simulink model "sl_ControlRobotReal_RRR"  (R2016b)
settings: Solver=ode45  StartTime=0.0  StopTime=t_sim  MaxStep=1e-3  RelTol=1e-3  EnableMultiTasking=on
values from neighbouring files (symbols this model uses):
  Kp1 = 1652.2*Ti1    (= 594.792)    [controladorPID.m]
  Kp2 = 5227.8*Ti2    (= 2091.12)    [controladorPID.m]
  Kp3 = 2761.4*Ti3    (= 994.104)    [controladorPID.m]
  n_ptos = 4    [pruebasCONTROL.m]
  R1 = 50    [modDinamico_Inverso_Ideal_CR.m]    (also in modDinamico_Inverso_Ideal_SR.m = 1; modDinamico_Inverso_Real_CR.m; modDinamico_Inverso_Real_SR.m = 1; pruebasCONTROL.m = 1)
  R2 = 30    [modDinamico_Inverso_Ideal_CR.m]    (also in modDinamico_Inverso_Ideal_SR.m = 1; modDinamico_Inverso_Real_CR.m; modDinamico_Inverso_Real_SR.m = 1; pruebasCONTROL.m = 1)
  R3 = 15    [modDinamico_Inverso_Ideal_CR.m]    (also in modDinamico_Inverso_Ideal_SR.m = 1; modDinamico_Inverso_Real_CR.m; modDinamico_Inverso_Real_SR.m = 1; pruebasCONTROL.m = 1)
  t_init_tray = 2    [pruebasCONTROL.m]
  t_mov = 1    [pruebasCONTROL.m]
  Td1 = (0.18^2)/(0.18*2)    (= 0.09)    [controladorPID.m]
  Td2 = (0.2^2)/(0.2*2)    (= 0.1)    [controladorPID.m]
  Td3 = (0.18^2)/(0.18*2)    (= 0.09)    [controladorPID.m]
  Ti1 = 2*0.18    (= 0.36)    [controladorPID.m]
  Ti2 = 2*0.2    (= 0.4)    [controladorPID.m]
  Ti3 = 2*0.18    (= 0.36)    [controladorPID.m]
  Tm = 0.001    [controladorPD.m]    (also in pruebasCONTROL.m)
  XYZ_fin = CinematicaDirecta([pi/2;pi/3;-pi/3])    [pruebasCONTROL.m]
  XYZ_init = CinematicaDirecta([q1_init;q2_init;q3_init])    [pruebasCONTROL.m]
undefined symbols (not defined in the file or in its folder): XYZ_med
undefined symbols (not defined in the file): q1_init, q2_init, q3_init
settings Model: ExtModeTrigMode=oneshot  ExtModeArmWhenConnect=off  Creator=mortega  LastModifiedBy=marrcogrova
settings DataIOCC: SaveFormat=Array  SignalLoggingSaveFormat=ModelDataLogs
settings OptimizationCC: BlockReduction=off  BooleanDataType=off  ExpressionDepthLimit=2147483647  InitFltsAndDblsToZero=on  LifeSpan=inf
settings DebuggingCC: SaveWithParameterizedLinksMsg=none  UnderspecifiedInitializationDetection=Classic  MergeDetectMultiDrivingBlocksExec=none  SignalResolutionControl=TryResolveAllWithWarning  MultiTaskDSMMsg=warning  MultiTaskCondExecSysMsg=none  FcnCallInpInsideContextMsg=warning  StateNameClashWarn=warning  SFUnexpectedBacktrackingDiag=warning  SFNoUnconditionalDefaultTransitionDiag=warning  SFExecutionAtInitializationDiag=none
settings HardwareCC: ProdBitPerPointer=32  ProdBitPerSizeT=32  ProdBitPerPtrDiffT=32  ProdLargestAtomicFloat=None  ProdIntDivRoundTo=Undefined  ProdEndianess=Unspecified  ProdWordSize=32  ProdHWDeviceType=32-bit Generic  TargetBitPerLong=64  TargetBitPerPointer=64  TargetBitPerSizeT=64  TargetBitPerPtrDiffT=64  TargetLongLongMode=on  TargetIntDivRoundTo=Zero  TargetEndianess=LittleEndian  TargetWordSize=64  TargetHWDeviceType=MATLAB Host  ProdEqTarget=off
settings ModelReferenceCC: PropagateSignalLabelsOutOfModel=off
settings GRTTargetCC: TargetFcnLib=ansi_tfl_tmw.mat  TargetLangStandard=C89/C90 (ANSI)  CombineOutputUpdateFcns=off  GRTInterface=on
settings ConfigComp: CovMetricSettings=dw  CovHtmlReporting=on  CovSaveCumulativeToWorkspaceVar=on  CovSaveSingleToWorkspaceVar=on  CovExternalEMLEnable=off

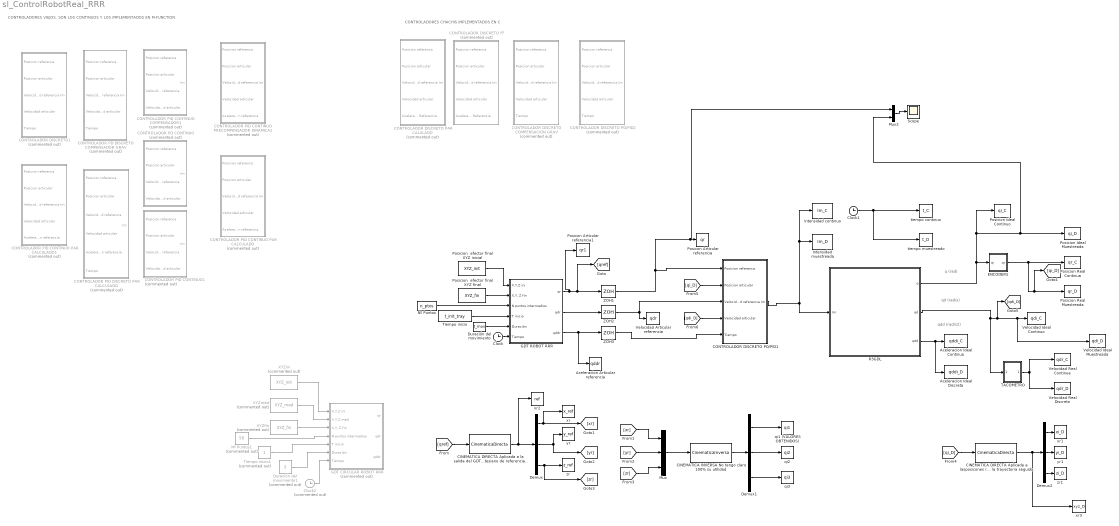
== system sl_ControlRobotReal_RRR ==
  note: CONTROLADORES VIEJOS.
      | SON LOS CONTINUOS Y LOS IMPLEMENTADOS EN M-FUNCTION
  note: q (rad)
  note: qd (rad/s)
  note: qdd (rad/s2)
  note: CONTROLADORES CHACHIS IMPLEMENTADOS EN C
  Aceleracion Articular referencia : ToWorkspace  VariableName=qddr  SampleTime=Tm
  Aceleracion Ideal Continua : ToWorkspace  VariableName=qddi_C  SampleTime=-1
  Aceleracion Ideal Discreta : ToWorkspace  VariableName=qddi_D  SampleTime=Tm
  CINEMATICA DIRECTA Aplicada a la salida del GDT para conocer la trayectoria en el plano cartesiano de referencia.. : MATLABFcn  MATLABFcn=CinematicaDirecta  OutputDimensions=3
  CINEMATICA DIRECTA Aplicada a lasposicones recogidas del robot para concer la trayectoria seguida. : MATLABFcn  MATLABFcn=CinematicaDirecta  OutputDimensions=3
  CINEMATICA INVERSA No tengo claro 100% su utilidad : MATLABFcn  MATLABFcn=CinematicaInversa  OutputDimensions=3
  CONTROLADOR DISCRETO COMPENSACION GRAV : Subsystem  Commented=on
  CONTROLADOR DISCRETO FF : Subsystem  Commented=on
  CONTROLADOR DISCRETO PAR CALULADO : Subsystem  Commented=on
  CONTROLADOR DISCRETO PD/PID1 : Subsystem
  CONTROLADOR DISCRETO PD/PID2 : Subsystem  Commented=on
  CONTROLADOR DISCRETO1 : Subsystem  Commented=on
  CONTROLADOR PD CONTINUO : Subsystem  Commented=on
  CONTROLADOR PD DISCRETO COMPENSADOR GRAV : Subsystem  Commented=on
  CONTROLADOR PID CONTINUO COMPENSADOR1 : Subsystem  Commented=on
  CONTROLADOR PID CONTINUO PAR CALCULADO : Subsystem  Commented=on
  CONTROLADOR PID CONTINUO PAR CALCULADO1 : Subsystem  Commented=on
  CONTROLADOR PID CONTINUO PRECOMPENSADOR DINAMICA2 : Subsystem  Commented=on
  CONTROLADOR PID CONTINUO1 : Subsystem  Commented=on
  "CONTROLADOR PID DISCRETO PAR CALCULADO " : Subsystem  Commented=on
  "Clock " : Clock
  Clock1 : Clock
  Clock2 : Clock  Commented=on
  Demux : Demux  Outputs=3
  Demux1 : Demux  Outputs=3
  Demux2 : Demux  Outputs=3
  Duración del movimiento : Constant  Value=t_mov
  Duración del movimiento1 : Constant  Commented=on  Value=3
  ENCODERS : Subsystem
  GDT CIRCULAR ROBOT RRR : Subsystem  Commented=on
  GDT ROBOT RRR : Subsystem
  Intensidad continuo : ToWorkspace  VariableName=Im_C  SampleTime=-1
  "Intensidad muestreada " : ToWorkspace  VariableName=Im_D  SampleTime=Tm
  Mux : Mux  Inputs=3
  Mux2 : Mux  Inputs=2
  Nº Puntos : Constant  Value=n_ptos
  Nº Puntos1 : Constant  Commented=on  Value=50
  Posicion  efector final XYZ final : Constant  Value=XYZ_fin
  Posicion  efector final XYZ inicial : Constant  Value=XYZ_init
  Posicion Ideal Continuo : ToWorkspace  VariableName=qi_C  SampleTime=-1
  Posicion Ideal Muestreada : ToWorkspace  VariableName=qi_D  SampleTime=Tm
  Posicion Real Continua : ToWorkspace  VariableName=qr_C  SampleTime=-1
  Posicion Real Muestreada : ToWorkspace  VariableName=qr_D  SampleTime=Tm
  Posicon Articular referencia : ToWorkspace  VariableName=qr  SampleTime=Tm
  Posicon Articular referencia1 : ToWorkspace  VariableName=qr1  SampleTime=Tm
  R3GDL : Subsystem  mask(Control y Programación de Robots (4 GIERM)){NGrupo=11, q1_ini=q1_init, q2_ini=q2_init, q3_ini=q3_init, Bl_q1=off, Bl_q2=off, Bl_q3=off, AccionamientoDirecto=on}
      mask prompts: NGrupo "Nº de GRUPO"; q1_ini "q1 inicial  (rad)"; q2_ini "q2 inicial (rad)"; q3_ini "q3_inicial (rad)"; Bl_q1 "Bloqueo q1"; Bl_q2 "Bloqueo q2"; Bl_q3 "Bloqueo q3"; AccionamientoDirecto "Accionamiento directo"
      mask help: Robot de 3 grados de libertad RRR
      mask Display:
      | image(imread('R3GDL_RRR.JPG'));
      | port_label('output', 1, 'q');
      | port_label('output', 2, 'qd');
      | port_label('output', 3, 'qdd');
      | port_label('input', 1, 'Im')
  Scope : Scope
  TACOMETRO : Subsystem
  Tiempo inicio : Constant  Value=t_init_tray
  Tiempo inicio1 : Constant  Commented=on
  Velocidad Articular referencia : ToWorkspace  VariableName=qdr  SampleTime=Tm
  Velocidad Ideal Continuo : ToWorkspace  VariableName=qdi_C  SampleTime=-1
  Velocidad Ideal Muestreada : ToWorkspace  VariableName=qdi_D  SampleTime=Tm
  Velocidad Real Continua : ToWorkspace  VariableName=qdr_C  SampleTime=-1
  Velocidad Real Discreto : ToWorkspace  VariableName=qdr_D  SampleTime=Tm
  XYZfin : Constant  Commented=on  Value=XYZ_fin
  XYZini : Constant  Commented=on  Value=XYZ_init
  XYZmed : Constant  Commented=on  Value=XYZ_med
  "ZOH1 " : ZeroOrderHold  SampleTime=10*Tm
  ZOH2 : ZeroOrderHold  SampleTime=10*Tm
  ZOH3 : ZeroOrderHold  SampleTime=10*Tm
  qi1 (VALORES OBTENIDOS) : ToWorkspace  VariableName=qi1  SampleTime=-1
  "qi2 " : ToWorkspace  VariableName=qi2  SampleTime=-1
  "qi3 " : ToWorkspace  VariableName=qi3  SampleTime=-1
  tiempo muestreado : ToWorkspace  VariableName=t_D  SampleTime=Tm
  tiempo continuo : ToWorkspace  VariableName=t_C  SampleTime=-1
  xr : ToWorkspace  VariableName=x_ref  SampleTime=-1
  xr1 : ToWorkspace  VariableName=xi_D  SampleTime=-1
  xr2 : ToWorkspace  VariableName=ref  SampleTime=Tm
  xr3 : ToWorkspace  VariableName=xyz_D  SampleTime=Tm
  yr : ToWorkspace  VariableName=y_ref  SampleTime=-1
  yr1 : ToWorkspace  VariableName=yi_D  SampleTime=-1
  zr : ToWorkspace  VariableName=z_ref  SampleTime=-1
  zr1 : ToWorkspace  VariableName=zi_D  SampleTime=-1
  wires:
  TACOMETRO/1(qdr) -> Velocidad Real Continua/1, Velocidad Real Discreto/1
  Clock1/1 -> tiempo continuo/1, tiempo muestreado/1
  R3GDL/3(qdd) -> Aceleracion Ideal Continua/1, Aceleracion Ideal Discreta/1
  Demux1/2 -> "qi2 "/1
  Demux/3 -> [zr], zr/1
  Demux1/1 -> qi1 (VALORES OBTENIDOS)/1
  [yr] -> Mux/2
  Mux/1 -> CINEMATICA INVERSA No tengo claro 100% su utilidad/1
  Demux/1 -> xr/1, [xr]
  CINEMATICA INVERSA No tengo claro 100% su utilidad/1 -> Demux1/1
  Demux1/3 -> "qi3 "/1
  [qref] -> CINEMATICA DIRECTA Aplicada a la salida del GDT para conocer la trayectoria en el plano cartesiano de referencia../1
  Demux/2 -> [yr], yr/1
  GDT ROBOT RRR/1(qr) -> Posicon Articular referencia1/1, "ZOH1 "/1, [qref]
  [xr] -> Mux/1
  [zr] -> Mux/3
  Demux2/3 -> zr1/1
  [qi_D] -> CINEMATICA DIRECTA Aplicada a lasposicones recogidas del robot para concer la trayectoria seguida./1
  Demux2/1 -> xr1/1
  Demux2/2 -> yr1/1
  GDT ROBOT RRR/3(qddr) -> ZOH3/1, Aceleracion Articular referencia/1
  GDT ROBOT RRR/2(qdr) -> ZOH2/1
  ZOH2/1 -> CONTROLADOR DISCRETO PD/PID1/3("Velocidad referencia "), Velocidad Articular referencia/1
  Mux2/1 -> Scope/1
  CINEMATICA DIRECTA Aplicada a la salida del GDT para conocer la trayectoria en el plano cartesiano de referencia../1 -> xr2/1, Demux/1
  CINEMATICA DIRECTA Aplicada a lasposicones recogidas del robot para concer la trayectoria seguida./1 -> xr3/1, Demux2/1
  "ZOH1 "/1 -> CONTROLADOR DISCRETO PD/PID1/1(Posicion referenca), Mux2/1, Posicon Articular referencia/1
  [qi_D] -> CONTROLADOR DISCRETO PD/PID1/2(Posicion articular)
  [qdi_D] -> CONTROLADOR DISCRETO PD/PID1/4(Velocidad articular)
  ZOH3/1 -> CONTROLADOR DISCRETO PD/PID1/5(Tiempo)
  CONTROLADOR DISCRETO PD/PID1/1(Im) -> "Intensidad muestreada "/1, Intensidad continuo/1, R3GDL/1(Im)
  R3GDL/2(qd) -> TACOMETRO/1(qdi), [qdi_D], Velocidad Ideal Muestreada/1, Velocidad Ideal Continuo/1
  R3GDL/1(q) -> Mux2/2, Posicion Ideal Muestreada/1, Posicion Ideal Continuo/1, ENCODERS/1(qi)
  ENCODERS/1(qr) -> Posicion Real Continua/1, [qi_D], Posicion Real Muestreada/1
  "Clock "/1 -> GDT ROBOT RRR/6(Tiempo)
  Posicion  efector final XYZ inicial/1 -> GDT ROBOT RRR/1(X,Y,Z ini)
  Posicion  efector final XYZ final/1 -> GDT ROBOT RRR/2("X,Y, Z fin")
  Nº Puntos/1 -> GDT ROBOT RRR/3(N puntos intermedios)
  Tiempo inicio/1 -> GDT ROBOT RRR/4(T inicio)
  Duración del movimiento/1 -> GDT ROBOT RRR/5(Duración)
  Clock2/1 -> GDT CIRCULAR ROBOT RRR/7(Tiempo)
  Duración del movimiento1/1 -> GDT CIRCULAR ROBOT RRR/6(Duración)
  Tiempo inicio1/1 -> GDT CIRCULAR ROBOT RRR/5(T inicio)
  Nº Puntos1/1 -> GDT CIRCULAR ROBOT RRR/4(N puntos intermedios)
  XYZfin/1 -> GDT CIRCULAR ROBOT RRR/3("X,Y, Z fin")
  XYZini/1 -> GDT CIRCULAR ROBOT RRR/1(X,Y,Z ini)
  XYZmed/1 -> GDT CIRCULAR ROBOT RRR/2("X,Y,Z med ")

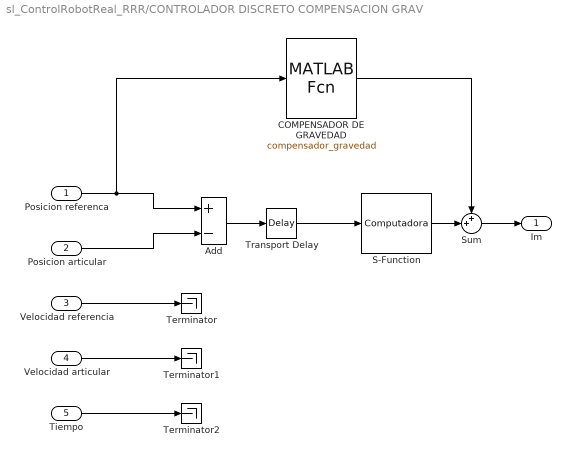
== system sl_ControlRobotReal_RRR/CONTROLADOR DISCRETO COMPENSACION GRAV ==
  Posicion referenca : Inport
  Posicion articular : Inport  Port=2
  "Velocidad referencia " : Inport  Port=3
  Velocidad articular : Inport  Port=4
  Tiempo : Inport  Port=5
  Add : Sum  Inputs=+-
  COMPENSADOR DE GRAVEDAD : MATLABFcn  MATLABFcn=compensador_gravedad  OutputDimensions=3
  S-Function : S-Function  FunctionName=Computadora  Parameters=Tm  SFunctionDeploymentMode=off  EnableBusSupport=off
  Sum : Sum  Inputs=++|
  Terminator : Terminator
  Terminator1 : Terminator
  Terminator2 : Terminator
  Transport Delay : TransportDelay  DelayTime=[1e-28;1e-28;1e-28]
  Im : Outport
  wires:
  "Velocidad referencia "/1 -> Terminator/1
  Posicion articular/1 -> Add/2
  Velocidad articular/1 -> Terminator1/1
  Tiempo/1 -> Terminator2/1
  Posicion referenca/1 -> COMPENSADOR DE GRAVEDAD/1, Add/1
  Add/1 -> Transport Delay/1
  Transport Delay/1 -> S-Function/1
  S-Function/1 -> Sum/2
  Sum/1 -> Im/1
  COMPENSADOR DE GRAVEDAD/1 -> Sum/1

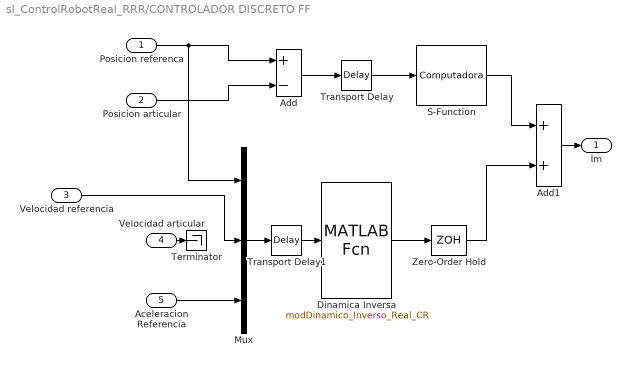
== system sl_ControlRobotReal_RRR/CONTROLADOR DISCRETO FF ==
  Posicion referenca : Inport
  Posicion articular : Inport  Port=2
  "Velocidad referencia " : Inport  Port=3
  Velocidad articular : Inport  Port=4
  "Aceleracion Referencia " : Inport  Port=5
  Add : Sum  Inputs=+-
  Add1 : Sum
  Dinamica Inversa : MATLABFcn  MATLABFcn=modDinamico_Inverso_Real_CR  OutputDimensions=3
  Mux : Mux  Inputs=3
  S-Function : S-Function  FunctionName=Computadora  Parameters=Tm  SFunctionDeploymentMode=off  EnableBusSupport=off
  Terminator : Terminator
  Transport Delay : TransportDelay  DelayTime=[1e-18;1e-18;1e-18]
  Transport Delay1 : TransportDelay  DelayTime=[1e-18;1e-18;1e-18;1e-18;1e-18;1e-18;1e-18;1e-18;1e-18]
  Zero-Order Hold : ZeroOrderHold  SampleTime=Tm
  Im : Outport
  wires:
  "Velocidad referencia "/1 -> Mux/2
  Posicion articular/1 -> Add/2
  "Aceleracion Referencia "/1 -> Mux/3
  Posicion referenca/1 -> Mux/1, Add/1
  Add/1 -> Transport Delay/1
  Transport Delay/1 -> S-Function/1
  S-Function/1 -> Add1/1
  Add1/1 -> Im/1
  Transport Delay1/1 -> Dinamica Inversa/1
  Mux/1 -> Transport Delay1/1
  Dinamica Inversa/1 -> Zero-Order Hold/1
  Zero-Order Hold/1 -> Add1/2
  Velocidad articular/1 -> Terminator/1

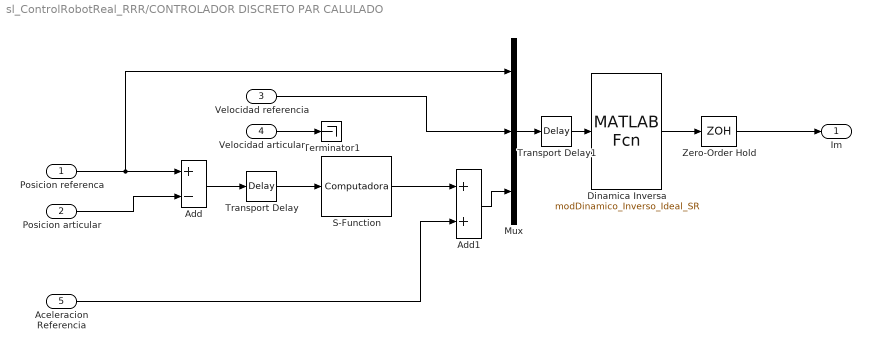
== system sl_ControlRobotReal_RRR/CONTROLADOR DISCRETO PAR CALULADO ==
  Posicion referenca : Inport
  Posicion articular : Inport  Port=2
  "Velocidad referencia " : Inport  Port=3
  Velocidad articular : Inport  Port=4
  "Aceleracion Referencia " : Inport  Port=5
  Add : Sum  Inputs=+-
  Add1 : Sum
  Dinamica Inversa : MATLABFcn  MATLABFcn=modDinamico_Inverso_Ideal_SR  OutputDimensions=3
  Mux : Mux  Inputs=3
  S-Function : S-Function  FunctionName=Computadora  Parameters=Tm  SFunctionDeploymentMode=off  EnableBusSupport=off
  Terminator1 : Terminator
  Transport Delay : TransportDelay  DelayTime=[1e-18;1e-18;1e-18]
  Transport Delay1 : TransportDelay  DelayTime=[1e-18;1e-18;1e-18;1e-18;1e-18;1e-18;1e-18;1e-18;1e-18]
  Zero-Order Hold : ZeroOrderHold  SampleTime=Tm
  Im : Outport
  wires:
  "Velocidad referencia "/1 -> Mux/2
  "Aceleracion Referencia "/1 -> Add1/2
  Transport Delay1/1 -> Dinamica Inversa/1
  Mux/1 -> Transport Delay1/1
  Dinamica Inversa/1 -> Zero-Order Hold/1
  Zero-Order Hold/1 -> Im/1
  Posicion articular/1 -> Add/2
  Posicion referenca/1 -> Mux/1, Add/1
  Add/1 -> Transport Delay/1
  Transport Delay/1 -> S-Function/1
  S-Function/1 -> Add1/1
  Add1/1 -> Mux/3
  Velocidad articular/1 -> Terminator1/1

== system sl_ControlRobotReal_RRR/CONTROLADOR DISCRETO PD//PID1 ==
  Posicion referenca : Inport
  Posicion articular : Inport  Port=2
  "Velocidad referencia " : Inport  Port=3
  Velocidad articular : Inport  Port=4
  Tiempo : Inport  Port=5
  Add : Sum  Inputs=+-
  S-Function : S-Function  FunctionName=Computadora  Parameters=Tm  SFunctionDeploymentMode=off  EnableBusSupport=off
  Terminator : Terminator
  Terminator1 : Terminator
  Terminator2 : Terminator
  Transport Delay : TransportDelay  DelayTime=[1e-28;1e-28;1e-28]
  Im : Outport
  wires:
  "Velocidad referencia "/1 -> Terminator/1
  Posicion articular/1 -> Add/2
  Velocidad articular/1 -> Terminator1/1
  Tiempo/1 -> Terminator2/1
  Posicion referenca/1 -> Add/1
  Add/1 -> Transport Delay/1
  Transport Delay/1 -> S-Function/1
  S-Function/1 -> Im/1

== system sl_ControlRobotReal_RRR/CONTROLADOR DISCRETO PD//PID2 ==
  Posicion referenca : Inport
  Posicion articular : Inport  Port=2
  "Velocidad referencia " : Inport  Port=3
  Velocidad articular : Inport  Port=4
  Tiempo : Inport  Port=5
  Add : Sum  Inputs=+-
  S-Function : S-Function  FunctionName=Computadora  Parameters=Tm  SFunctionDeploymentMode=off  EnableBusSupport=off
  Terminator : Terminator
  Terminator1 : Terminator
  Terminator2 : Terminator
  Transport Delay : TransportDelay  DelayTime=[1e-28;1e-28;1e-28]
  Im : Outport
  wires:
  "Velocidad referencia "/1 -> Terminator/1
  Posicion articular/1 -> Add/2
  Velocidad articular/1 -> Terminator1/1
  Tiempo/1 -> Terminator2/1
  Posicion referenca/1 -> Add/1
  Add/1 -> Transport Delay/1
  Transport Delay/1 -> S-Function/1
  S-Function/1 -> Im/1

== system sl_ControlRobotReal_RRR/CONTROLADOR DISCRETO1 ==
  Posicion referenca : Inport
  Posicion articular : Inport  Port=2
  "Velocidad referencia " : Inport  Port=3
  Velocidad articular : Inport  Port=4
  Tiempo : Inport  Port=5
  CONTROL : MATLABFcn  MATLABFcn=controladorPD  OutputDimensions=3
  MANTENEDOR DE ORDEN 0 (Se usa para muestrear la salida continua de la funcion interpretada continua) : ZeroOrderHold  SampleTime=Tm
  Mux1 : Mux  Inputs=5
  Im : Outport
  wires:
  "Velocidad referencia "/1 -> Mux1/3
  MANTENEDOR DE ORDEN 0 (Se usa para muestrear la salida continua de la funcion interpretada continua)/1 -> Im/1
  Posicion articular/1 -> Mux1/2
  Velocidad articular/1 -> Mux1/4
  Tiempo/1 -> Mux1/5
  Posicion referenca/1 -> Mux1/1
  Mux1/1 -> CONTROL/1
  CONTROL/1 -> MANTENEDOR DE ORDEN 0 (Se usa para muestrear la salida continua de la funcion interpretada continua)/1

== system sl_ControlRobotReal_RRR/CONTROLADOR PD CONTINUO ==
  Posicion referenca : Inport
  Posicion articular : Inport  Port=2
  "Velocidad referencia " : Inport  Port=3
  Velocidad articular : Inport  Port=4
  Add : Sum  Inputs=+-
  Add1 : Sum  Inputs=+-
  Add2 : Sum
  Kp : Gain  Gain=[Kp1;Kp2;Kp3]
  Kp*Td : Gain  Gain=[Kp1*Td1;Kp2*Td2;Kp3*Td3]
  MANTENEDOR DE ORDEN 0 (Se usa para muestrear la salida continua de la funcion interpretada continua) : ZeroOrderHold  SampleTime=Tm
  Im : Outport
  wires:
  "Velocidad referencia "/1 -> Add1/1
  MANTENEDOR DE ORDEN 0 (Se usa para muestrear la salida continua de la funcion interpretada continua)/1 -> Im/1
  Add2/1 -> MANTENEDOR DE ORDEN 0 (Se usa para muestrear la salida continua de la funcion interpretada continua)/1
  Posicion articular/1 -> Add/2
  Velocidad articular/1 -> Add1/2
  Posicion referenca/1 -> Add/1
  Add/1 -> Kp/1
  Add1/1 -> Kp*Td/1
  Kp*Td/1 -> Add2/2
  Kp/1 -> Add2/1

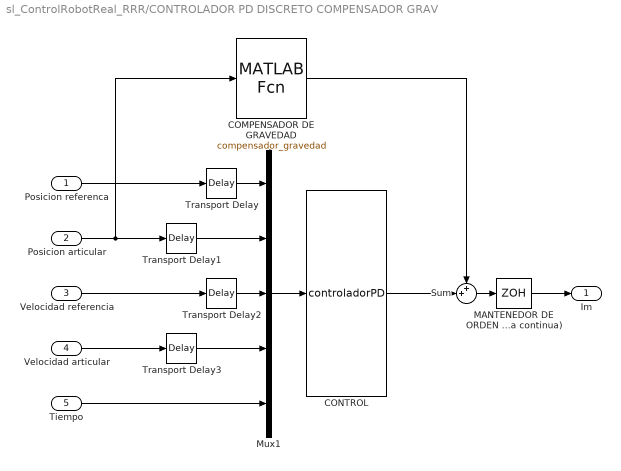
== system sl_ControlRobotReal_RRR/CONTROLADOR PD DISCRETO COMPENSADOR GRAV ==
  Posicion referenca : Inport
  Posicion articular : Inport  Port=2
  "Velocidad referencia " : Inport  Port=3
  Velocidad articular : Inport  Port=4
  Tiempo : Inport  Port=5
  COMPENSADOR DE GRAVEDAD : MATLABFcn  MATLABFcn=compensador_gravedad
  CONTROL : MATLABFcn  MATLABFcn=controladorPD  OutputDimensions=3
  MANTENEDOR DE ORDEN 0 (Se usa para muestrear la salida continua de la funcion interpretada continua) : ZeroOrderHold  SampleTime=Tm
  Mux1 : Mux  Inputs=5
  Sum : Sum  Inputs=++|
  Transport Delay{,1..3} (4 alike) : TransportDelay  DelayTime=1e-18  InitialOutput=[1.8;0;1.2]
  Im : Outport
  wires:
  MANTENEDOR DE ORDEN 0 (Se usa para muestrear la salida continua de la funcion interpretada continua)/1 -> Im/1
  Posicion articular/1 -> COMPENSADOR DE GRAVEDAD/1, Transport Delay1/1
  COMPENSADOR DE GRAVEDAD/1 -> Sum/1
  CONTROL/1 -> Sum/2
  Sum/1 -> MANTENEDOR DE ORDEN 0 (Se usa para muestrear la salida continua de la funcion interpretada continua)/1
  Tiempo/1 -> Mux1/5
  Mux1/1 -> CONTROL/1
  Posicion referenca/1 -> Transport Delay/1
  "Velocidad referencia "/1 -> Transport Delay2/1
  Velocidad articular/1 -> Transport Delay3/1
  Transport Delay/1 -> Mux1/1
  Transport Delay1/1 -> Mux1/2
  Transport Delay2/1 -> Mux1/3
  Transport Delay3/1 -> Mux1/4

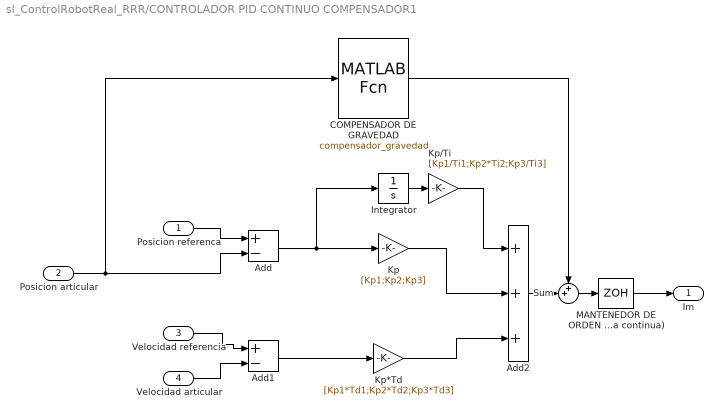
== system sl_ControlRobotReal_RRR/CONTROLADOR PID CONTINUO COMPENSADOR1 ==
  Posicion referenca : Inport
  Posicion articular : Inport  Port=2
  "Velocidad referencia " : Inport  Port=3
  Velocidad articular : Inport  Port=4
  Add : Sum  Inputs=+-
  Add1 : Sum  Inputs=+-
  Add2 : Sum  Inputs=+++
  COMPENSADOR DE GRAVEDAD : MATLABFcn  MATLABFcn=compensador_gravedad
  Integrator : Integrator
  Kp : Gain  Gain=[Kp1;Kp2;Kp3]
  Kp*Td : Gain  Gain=[Kp1*Td1;Kp2*Td2;Kp3*Td3]
  Kp/Ti : Gain  Gain=[Kp1/Ti1;Kp2*Ti2;Kp3/Ti3]
  MANTENEDOR DE ORDEN 0 (Se usa para muestrear la salida continua de la funcion interpretada continua) : ZeroOrderHold  SampleTime=Tm
  Sum : Sum  Inputs=++|
  Im : Outport
  wires:
  "Velocidad referencia "/1 -> Add1/1
  MANTENEDOR DE ORDEN 0 (Se usa para muestrear la salida continua de la funcion interpretada continua)/1 -> Im/1
  Posicion articular/1 -> COMPENSADOR DE GRAVEDAD/1, Add/2
  Velocidad articular/1 -> Add1/2
  Posicion referenca/1 -> Add/1
  Add/1 -> Integrator/1, Kp/1
  Integrator/1 -> Kp/Ti/1
  Add1/1 -> Kp*Td/1
  Kp/Ti/1 -> Add2/1
  Kp/1 -> Add2/2
  Kp*Td/1 -> Add2/3
  COMPENSADOR DE GRAVEDAD/1 -> Sum/1
  Add2/1 -> Sum/2
  Sum/1 -> MANTENEDOR DE ORDEN 0 (Se usa para muestrear la salida continua de la funcion interpretada continua)/1

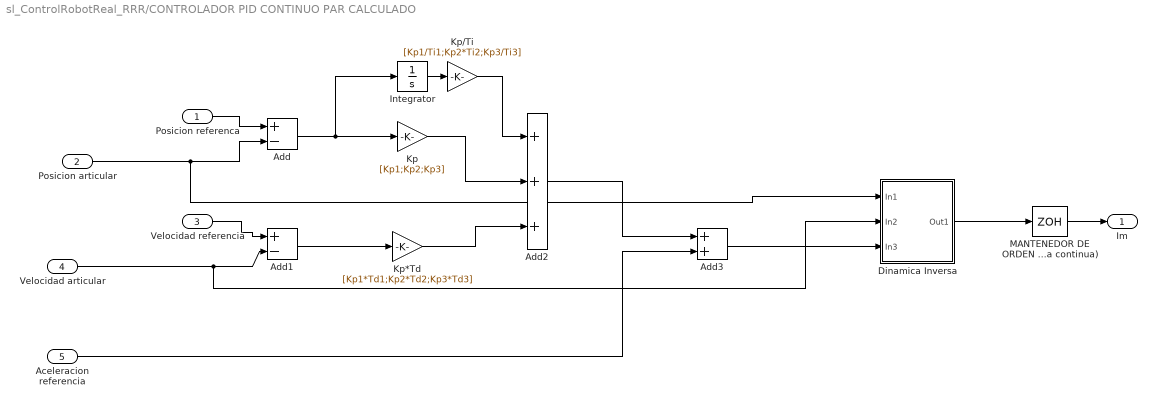
== system sl_ControlRobotReal_RRR/CONTROLADOR PID CONTINUO PAR CALCULADO ==
  Posicion referenca : Inport
  Posicion articular : Inport  Port=2
  "Velocidad referencia " : Inport  Port=3
  Velocidad articular : Inport  Port=4
  Aceleracion referencia : Inport  Port=5
  Add : Sum  Inputs=+-
  Add1 : Sum  Inputs=+-
  Add2 : Sum  Inputs=+++
  Add3 : Sum
  "Dinamica Inversa " : Subsystem
  Integrator : Integrator
  Kp : Gain  Gain=[Kp1;Kp2;Kp3]
  Kp*Td : Gain  Gain=[Kp1*Td1;Kp2*Td2;Kp3*Td3]
  Kp/Ti : Gain  Gain=[Kp1/Ti1;Kp2*Ti2;Kp3/Ti3]
  MANTENEDOR DE ORDEN 0 (Se usa para muestrear la salida continua de la funcion interpretada continua) : ZeroOrderHold  SampleTime=Tm
  Im : Outport
  wires:
  "Velocidad referencia "/1 -> Add1/1
  MANTENEDOR DE ORDEN 0 (Se usa para muestrear la salida continua de la funcion interpretada continua)/1 -> Im/1
  Posicion articular/1 -> "Dinamica Inversa "/1(In1), Add/2
  Posicion referenca/1 -> Add/1
  Add/1 -> Integrator/1, Kp/1
  Integrator/1 -> Kp/Ti/1
  Add1/1 -> Kp*Td/1
  Kp/Ti/1 -> Add2/1
  Kp/1 -> Add2/2
  Kp*Td/1 -> Add2/3
  Velocidad articular/1 -> "Dinamica Inversa "/2(In2), Add1/2
  Add2/1 -> Add3/1
  Add3/1 -> "Dinamica Inversa "/3(In3)
  "Dinamica Inversa "/1(Out1) -> MANTENEDOR DE ORDEN 0 (Se usa para muestrear la salida continua de la funcion interpretada continua)/1
  Aceleracion referencia/1 -> Add3/2

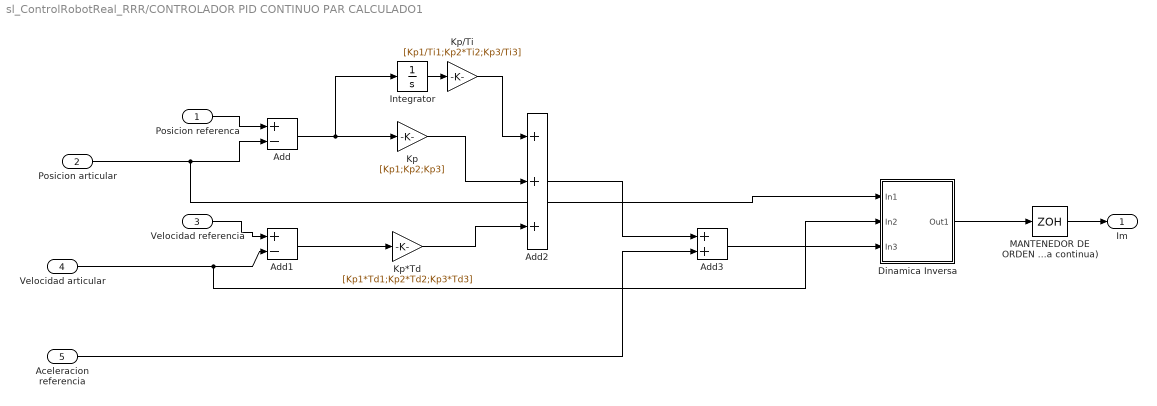
== system sl_ControlRobotReal_RRR/CONTROLADOR PID CONTINUO PAR CALCULADO1 ==
  Posicion referenca : Inport
  Posicion articular : Inport  Port=2
  "Velocidad referencia " : Inport  Port=3
  Velocidad articular : Inport  Port=4
  Aceleracion referencia : Inport  Port=5
  Add : Sum  Inputs=+-
  Add1 : Sum  Inputs=+-
  Add2 : Sum  Inputs=+++
  Add3 : Sum
  "Dinamica Inversa " : Subsystem
  Integrator : Integrator
  Kp : Gain  Gain=[Kp1;Kp2;Kp3]
  Kp*Td : Gain  Gain=[Kp1*Td1;Kp2*Td2;Kp3*Td3]
  Kp/Ti : Gain  Gain=[Kp1/Ti1;Kp2*Ti2;Kp3/Ti3]
  MANTENEDOR DE ORDEN 0 (Se usa para muestrear la salida continua de la funcion interpretada continua) : ZeroOrderHold  SampleTime=Tm
  Im : Outport
  wires:
  "Velocidad referencia "/1 -> Add1/1
  MANTENEDOR DE ORDEN 0 (Se usa para muestrear la salida continua de la funcion interpretada continua)/1 -> Im/1
  Posicion articular/1 -> "Dinamica Inversa "/1(In1), Add/2
  Posicion referenca/1 -> Add/1
  Add/1 -> Integrator/1, Kp/1
  Integrator/1 -> Kp/Ti/1
  Add1/1 -> Kp*Td/1
  Kp/Ti/1 -> Add2/1
  Kp/1 -> Add2/2
  Kp*Td/1 -> Add2/3
  Velocidad articular/1 -> "Dinamica Inversa "/2(In2), Add1/2
  Add2/1 -> Add3/1
  Add3/1 -> "Dinamica Inversa "/3(In3)
  "Dinamica Inversa "/1(Out1) -> MANTENEDOR DE ORDEN 0 (Se usa para muestrear la salida continua de la funcion interpretada continua)/1
  Aceleracion referencia/1 -> Add3/2

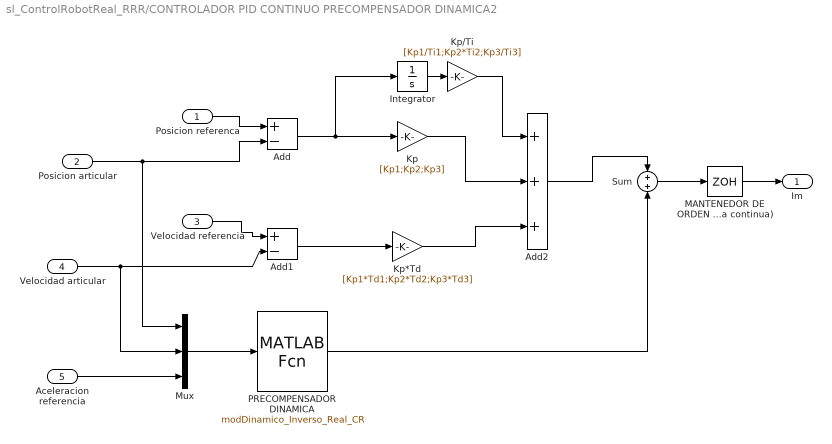
== system sl_ControlRobotReal_RRR/CONTROLADOR PID CONTINUO PRECOMPENSADOR DINAMICA2 ==
  Posicion referenca : Inport
  Posicion articular : Inport  Port=2
  "Velocidad referencia " : Inport  Port=3
  Velocidad articular : Inport  Port=4
  Aceleracion referencia : Inport  Port=5
  Add : Sum  Inputs=+-
  Add1 : Sum  Inputs=+-
  Add2 : Sum  Inputs=+++
  Integrator : Integrator
  Kp : Gain  Gain=[Kp1;Kp2;Kp3]
  Kp*Td : Gain  Gain=[Kp1*Td1;Kp2*Td2;Kp3*Td3]
  Kp/Ti : Gain  Gain=[Kp1/Ti1;Kp2*Ti2;Kp3/Ti3]
  MANTENEDOR DE ORDEN 0 (Se usa para muestrear la salida continua de la funcion interpretada continua) : ZeroOrderHold  SampleTime=Tm
  Mux : Mux  Inputs=3
  PRECOMPENSADOR DINAMICA : MATLABFcn  MATLABFcn=modDinamico_Inverso_Real_CR  OutputDimensions=3
  Sum : Sum
  Im : Outport
  wires:
  "Velocidad referencia "/1 -> Add1/1
  MANTENEDOR DE ORDEN 0 (Se usa para muestrear la salida continua de la funcion interpretada continua)/1 -> Im/1
  Posicion articular/1 -> Mux/1, Add/2
  Posicion referenca/1 -> Add/1
  Add/1 -> Integrator/1, Kp/1
  Integrator/1 -> Kp/Ti/1
  Add1/1 -> Kp*Td/1
  Kp/Ti/1 -> Add2/1
  Kp/1 -> Add2/2
  Kp*Td/1 -> Add2/3
  Sum/1 -> MANTENEDOR DE ORDEN 0 (Se usa para muestrear la salida continua de la funcion interpretada continua)/1
  Mux/1 -> PRECOMPENSADOR DINAMICA/1
  PRECOMPENSADOR DINAMICA/1 -> Sum/2
  Velocidad articular/1 -> Mux/2, Add1/2
  Aceleracion referencia/1 -> Mux/3
  Add2/1 -> Sum/1

== system sl_ControlRobotReal_RRR/CONTROLADOR PID CONTINUO1 ==
  Posicion referenca : Inport
  Posicion articular : Inport  Port=2
  "Velocidad referencia " : Inport  Port=3
  Velocidad articular : Inport  Port=4
  Add : Sum  Inputs=+-
  Add1 : Sum  Inputs=+-
  Add2 : Sum  Inputs=+++
  Integrator : Integrator  Commented=on  InitialCondition=[0;0;0]
  Kp : Gain  Gain=[Kp1;Kp2;Kp3]
  Kp*Td : Gain  Gain=[Kp1*Td1;Kp2*Td2;Kp3*Td3]
  Kp/Ti : Gain  Commented=on  Gain=[Kp1/Ti1;Kp2/Ti2;Kp3/Ti3]
  MANTENEDOR DE ORDEN 0 (Se usa para muestrear la salida continua de la funcion interpretada continua) : ZeroOrderHold  SampleTime=Tm
  Im : Outport
  wires:
  "Velocidad referencia "/1 -> Add1/1
  MANTENEDOR DE ORDEN 0 (Se usa para muestrear la salida continua de la funcion interpretada continua)/1 -> Im/1
  Add2/1 -> MANTENEDOR DE ORDEN 0 (Se usa para muestrear la salida continua de la funcion interpretada continua)/1
  Posicion articular/1 -> Add/2
  Velocidad articular/1 -> Add1/2
  Posicion referenca/1 -> Add/1
  Add/1 -> Integrator/1, Kp/1
  Integrator/1 -> Kp/Ti/1
  Add1/1 -> Kp*Td/1
  Kp/Ti/1 -> Add2/1
  Kp/1 -> Add2/2
  Kp*Td/1 -> Add2/3

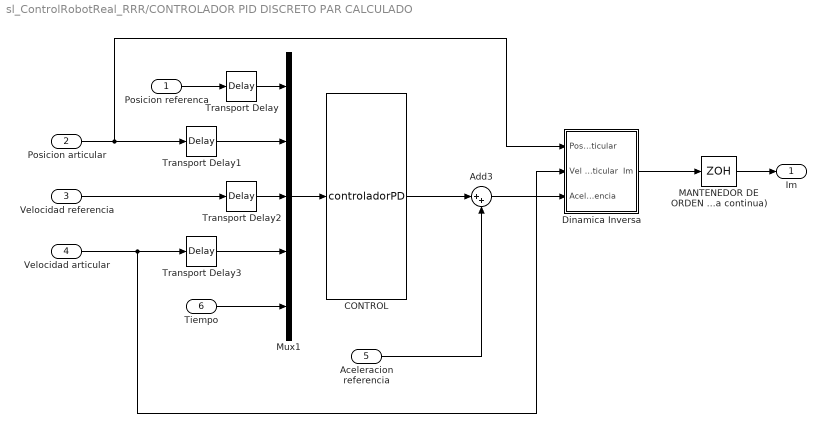
== system sl_ControlRobotReal_RRR/CONTROLADOR PID DISCRETO PAR CALCULADO  ==
  Posicion referenca : Inport
  Posicion articular : Inport  Port=2
  "Velocidad referencia " : Inport  Port=3
  Velocidad articular : Inport  Port=4
  Aceleracion referencia : Inport  Port=5
  Tiempo : Inport  Port=6
  Add3 : Sum  Inputs=|++
  CONTROL : MATLABFcn  MATLABFcn=controladorPD  OutputDimensions=3
  "Dinamica Inversa " : Subsystem
  MANTENEDOR DE ORDEN 0 (Se usa para muestrear la salida continua de la funcion interpretada continua) : ZeroOrderHold  SampleTime=Tm
  Mux1 : Mux  Inputs=5
  Transport Delay{,1..3} (4 alike) : TransportDelay  DelayTime=1e-18  InitialOutput=[1.8;0;1.2]
  Im : Outport
  wires:
  MANTENEDOR DE ORDEN 0 (Se usa para muestrear la salida continua de la funcion interpretada continua)/1 -> Im/1
  Add3/1 -> "Dinamica Inversa "/3(Acel referencia)
  "Dinamica Inversa "/1(Im) -> MANTENEDOR DE ORDEN 0 (Se usa para muestrear la salida continua de la funcion interpretada continua)/1
  Aceleracion referencia/1 -> Add3/2
  Posicion articular/1 -> "Dinamica Inversa "/1(Pos articular), Transport Delay1/1
  Tiempo/1 -> Mux1/5
  Mux1/1 -> CONTROL/1
  Posicion referenca/1 -> Transport Delay/1
  "Velocidad referencia "/1 -> Transport Delay2/1
  Velocidad articular/1 -> "Dinamica Inversa "/2(Vel articular), Transport Delay3/1
  Transport Delay/1 -> Mux1/1
  Transport Delay1/1 -> Mux1/2
  Transport Delay2/1 -> Mux1/3
  Transport Delay3/1 -> Mux1/4
  CONTROL/1 -> Add3/1

== system sl_ControlRobotReal_RRR/ENCODERS ==
  qi : Inport
  Demux : Demux  Outputs=3
  Mux2 : Mux  Inputs=3
  Quantizer (Encoder) : Quantizer  QuantizationInterval=2*pi/512/R1
  Quantizer (Encoder)1 : Quantizer  QuantizationInterval=2*pi/512/R2
  Quantizer (Encoder)2 : Quantizer  QuantizationInterval=2*pi/512/R3
  qr : Outport
  wires:
  Demux/2 -> Quantizer (Encoder)1/1
  Demux/1 -> Quantizer (Encoder)/1
  Quantizer (Encoder)1/1 -> Mux2/2
  Mux2/1 -> qr/1
  Quantizer (Encoder)2/1 -> Mux2/3
  Demux/3 -> Quantizer (Encoder)2/1
  qi/1 -> Demux/1
  Quantizer (Encoder)/1 -> Mux2/1

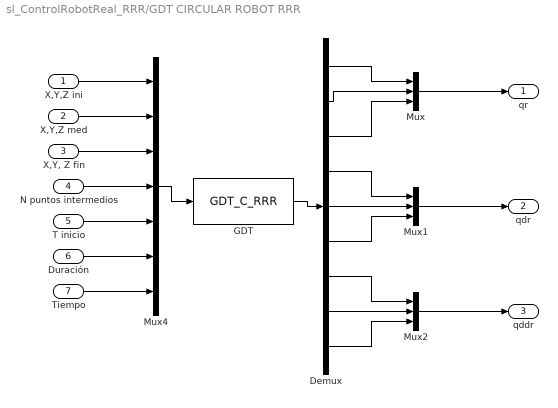
== system sl_ControlRobotReal_RRR/GDT CIRCULAR ROBOT RRR ==
  X,Y,Z ini : Inport
  "X,Y,Z med " : Inport  Port=2
  "X,Y, Z fin" : Inport  Port=3
  N puntos intermedios : Inport  Port=4
  T inicio : Inport  Port=5
  Duración : Inport  Port=6
  Tiempo : Inport  Port=7
  Demux : Demux  Outputs=9
  "GDT " : MATLABFcn  MATLABFcn=GDT_C_RRR  OutputDimensions=9
  Mux : Mux  Inputs=3
  Mux1 : Mux  Inputs=3
  Mux2 : Mux  Inputs=3
  Mux4 : Mux  Inputs=7
  qr : Outport
  qdr : Outport  Port=2
  qddr : Outport  Port=3
  wires:
  Mux4/1 -> "GDT "/1
  "GDT "/1 -> Demux/1
  Mux/1 -> qr/1
  Demux/1 -> Mux/1
  Demux/2 -> Mux/2
  Demux/3 -> Mux/3
  Demux/5 -> Mux1/2
  Demux/4 -> Mux1/1
  Demux/6 -> Mux1/3
  Mux1/1 -> qdr/1
  Demux/8 -> Mux2/2
  Mux2/1 -> qddr/1
  Demux/7 -> Mux2/1
  Demux/9 -> Mux2/3
  X,Y,Z ini/1 -> Mux4/1
  "X,Y,Z med "/1 -> Mux4/2
  "X,Y, Z fin"/1 -> Mux4/3
  N puntos intermedios/1 -> Mux4/4
  T inicio/1 -> Mux4/5
  Duración/1 -> Mux4/6
  Tiempo/1 -> Mux4/7

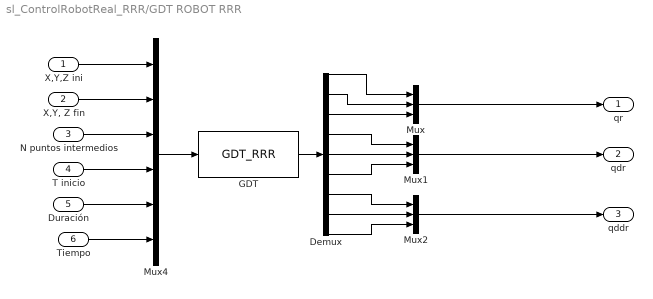
== system sl_ControlRobotReal_RRR/GDT ROBOT RRR ==
  X,Y,Z ini : Inport
  "X,Y, Z fin" : Inport  Port=2
  N puntos intermedios : Inport  Port=3
  T inicio : Inport  Port=4
  Duración : Inport  Port=5
  Tiempo : Inport  Port=6
  Demux : Demux  Outputs=9
  "GDT " : MATLABFcn  MATLABFcn=GDT_RRR  OutputDimensions=9
  Mux : Mux  Inputs=3
  Mux1 : Mux  Inputs=3
  Mux2 : Mux  Inputs=3
  Mux4 : Mux  Inputs=6
  qr : Outport
  qdr : Outport  Port=2
  qddr : Outport  Port=3
  wires:
  Mux4/1 -> "GDT "/1
  X,Y,Z ini/1 -> Mux4/1
  "X,Y, Z fin"/1 -> Mux4/2
  N puntos intermedios/1 -> Mux4/3
  T inicio/1 -> Mux4/4
  Duración/1 -> Mux4/5
  Tiempo/1 -> Mux4/6
  "GDT "/1 -> Demux/1
  Mux/1 -> qr/1
  Demux/1 -> Mux/1
  Demux/2 -> Mux/2
  Demux/3 -> Mux/3
  Demux/5 -> Mux1/2
  Demux/4 -> Mux1/1
  Demux/6 -> Mux1/3
  Mux1/1 -> qdr/1
  Demux/8 -> Mux2/2
  Mux2/1 -> qddr/1
  Demux/7 -> Mux2/1
  Demux/9 -> Mux2/3

== system sl_ControlRobotReal_RRR/R3GDL ==
  Im : Inport
  S-Function : S-Function  FunctionName=R3GDL_RRR  Parameters=[q1_ini; q2_ini; q3_ini]; [Bl_q1; Bl_q2; Bl_q3]; AccionamientoDirecto; NGrupo  SFunctionDeploymentMode=off  EnableBusSupport=off
  q : Outport
  qd : Outport  Port=2
  qdd : Outport  Port=3
  wires:
  Im/1 -> S-Function/1
  S-Function/1 -> q/1
  S-Function/2 -> qd/1
  S-Function/3 -> qdd/1

== system sl_ControlRobotReal_RRR/TACOMETRO ==
  qdi : Inport
  Add : Sum  Inputs=++|
  Add1 : Sum  Inputs=|++
  Add2 : Sum  Inputs=|++
  Demux : Demux  Outputs=3
  Mux2 : Mux  Inputs=3
  Uniform Random Number : UniformRandomNumber  Minimum=-(157/R1)*0.02  Maximum=(157/R1)*0.02  SampleTime=Tm
  Uniform Random Number1 : UniformRandomNumber  Minimum=-(157/R2)*0.02  Maximum=(157/R2)*0.02  SampleTime=Tm
  Uniform Random Number2 : UniformRandomNumber  Minimum=-(157/R3)*0.02  Maximum=(157/R3)*0.02  SampleTime=Tm
  qdr : Outport
  wires:
  Demux/2 -> Add1/1
  Add1/1 -> Mux2/2
  Add/1 -> Mux2/1
  Demux/1 -> Add/2
  Uniform Random Number1/1 -> Add1/2
  Add2/1 -> Mux2/3
  Uniform Random Number2/1 -> Add2/2
  Uniform Random Number/1 -> Add/1
  Demux/3 -> Add2/1
  Mux2/1 -> qdr/1
  qdi/1 -> Demux/1

== system sl_ControlRobotReal_RRR/CONTROLADOR PID CONTINUO PAR CALCULADO/Dinamica Inversa  ==
  In1 : Inport
  In2 : Inport  Port=2
  In3 : Inport  Port=3
  Mux : Mux  Inputs=3
  "PAR CALCULADO " : MATLABFcn  MATLABFcn=modDinamico_Inverso_Ideal_CR  OutputDimensions=3
  Out1 : Outport
  wires:
  "PAR CALCULADO "/1 -> Out1/1
  In2/1 -> Mux/2
  In1/1 -> Mux/1
  In3/1 -> Mux/3
  Mux/1 -> "PAR CALCULADO "/1

== system sl_ControlRobotReal_RRR/CONTROLADOR PID CONTINUO PAR CALCULADO1/Dinamica Inversa  ==
  In1 : Inport
  In2 : Inport  Port=2
  In3 : Inport  Port=3
  Mux : Mux  Inputs=3
  "PAR CALCULADO " : MATLABFcn  MATLABFcn=modDinamico_Inverso_Ideal_CR  OutputDimensions=3
  Out1 : Outport
  wires:
  "PAR CALCULADO "/1 -> Out1/1
  In2/1 -> Mux/2
  In1/1 -> Mux/1
  In3/1 -> Mux/3
  Mux/1 -> "PAR CALCULADO "/1

== system sl_ControlRobotReal_RRR/CONTROLADOR PID DISCRETO PAR CALCULADO /Dinamica Inversa  ==
  Pos articular : Inport
  Vel articular : Inport  Port=2
  Acel referencia : Inport  Port=3
  Mux : Mux  Inputs=3
  "PAR CALCULADO " : MATLABFcn  MATLABFcn=par_calculado  OutputDimensions=3
  Im : Outport
  wires:
  "PAR CALCULADO "/1 -> Im/1
  Vel articular/1 -> Mux/2
  Pos articular/1 -> Mux/1
  Acel referencia/1 -> Mux/3
  Mux/1 -> "PAR CALCULADO "/1
